simulink model "racing_wheel_lqr_observer"  (R2019b)
settings: Solver=FixedStepAuto  StartTime=0.0  StopTime=inf  FixedStep=0.01  RelTol=1e-3
values from neighbouring files (symbols this model uses):
  Kw = 1/(sys_dis.C*inv(eye(2) - sys_dis.A + sys_dis.B*K)*sys_dis.B)    [controller_LQR_tryout.m]
  P = double([SOL.P1;SOL.P2])    [controller_LQR_tryout.m]
  sys_dis = c2d(sys_con,Ts)    [controller_LQR_tryout.m]
  Ts = 0.02    [controller_LQR_tryout.m]
undefined symbols (not defined in the file or in its folder): K, K_int
libraries: sldrtlib x1
settings Model: EnablePacing=on  Creator=mandl  LastModifiedBy=mandl
settings SolverCC: AlgebraicLoopSolver=LineSearch

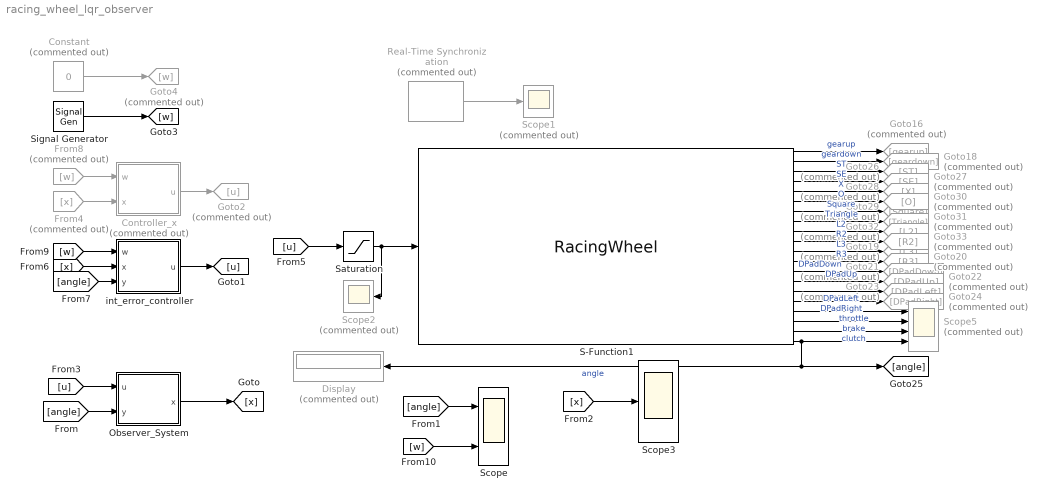
== system racing_wheel_lqr_observer ==
  Constant : Constant  Commented=on  Value=0
  Controller_x : Subsystem  Commented=on
  Display : Display  Commented=on
  From4 : From  Commented=on  GotoTag=x
  From8 : From  Commented=on  GotoTag=w
  Goto16 : Goto  Commented=on  GotoTag=gearup
  Goto18 : Goto  Commented=on  GotoTag=geardown
  Goto19 : Goto  Commented=on  GotoTag=L3
  Goto2 : Goto  Commented=on  GotoTag=u
  Goto20 : Goto  Commented=on  GotoTag=R3
  Goto21 : Goto  Commented=on  GotoTag=DPadDown
  Goto22 : Goto  Commented=on  GotoTag=DPadUp
  Goto23 : Goto  Commented=on  GotoTag=DPadLeft
  Goto24 : Goto  Commented=on  GotoTag=DPadRight
  Goto26 : Goto  Commented=on  GotoTag=ST
  Goto27 : Goto  Commented=on  GotoTag=SE
  Goto28 : Goto  Commented=on  GotoTag=X
  Goto29 : Goto  Commented=on  GotoTag=Square
  Goto30 : Goto  Commented=on  GotoTag=O
  Goto31 : Goto  Commented=on  GotoTag=Triangle
  Goto32 : Goto  Commented=on  GotoTag=L2
  Goto33 : Goto  Commented=on  GotoTag=R2
  Goto4 : Goto  Commented=on  GotoTag=w
  Observer_System : Subsystem
  Real-Time Synchronization : sldrtlib/Real-Time Synchronization  Commented=on  SampleTime=Ts  MaxMissedTicks=inf  ShowMissedTicks=on  YieldWhenWaiting=off
  S-Function1 : S-Function  FunctionName=RacingWheel  Parameters=Ts_FF  SFunctionModules=RacingWheel_wrapper  SFunctionDeploymentMode=off  EnableBusSupport=off  mask(Racing Wheel with Force Feedback){Ts_FF=Ts}
      mask prompts: Ts_FF "Constant Force-Feedback Sample Time"
      mask help: Interacts with the windows gaming API from UWP. The force feedback effect is constant over the user defined sampling time below.
      mask init:
      | val = [[.9  0.75 0.75 1 1 .9 .9 1]',[1 1 0.75 0.75 .9 .9 1 .9]'];try , sys = get_param(gcb,'SfunBuilderFcnName');if isempty(sys), sys = get_param(gcb,'FunctionName'); end,catch, sys = get_param(gcb,'FunctionName'); end
      mask Display:
      | plot(val(:,1),val(:,2)),disp(sys),
      | image('icon.png'),
      | port_label('input',1,'FF'),
      | port_label('output',1,'gearup'),
      | port_label('output',2,'geardown'),
      | port_label('output',3,'ST'),
      | port_label('output',4,'SE'),
      | port_label('output',5,'X'),
      | port_label('output',6,'O'),
      | port_label('output',7,'Square'),
      | port_label('output',8,'Triangle'),
      | port_label('output',9,'L2'),
      | port_label('output',10,'R2'),
      | port_label('output',11,'L3'),
      | port_label('output',12,'R3'),
      | port_label('output',13,'DPadDown'),
      | port_label('output',14,'DPadUp'),
      | port_label('output',15,'DPadLeft'),
      | port_label('output',16,'DPadRight'),
      | port_label('output',17,'throttle'),
      | port_label('output',18,'brake'),
      | port_label('output',19,'clutch'),
      | port_label('output',20,'angle')
  Saturation : Saturate  UpperLimit=1  LowerLimit=-1
  Scope : Scope  NumInputPorts=2
  Scope1 : Scope  Commented=on
  Scope2 : Scope  Commented=on
  Scope3 : Scope
  Scope5 : Scope  Commented=on  NumInputPorts=4
  Signal Generator : SignalGenerator  Amplitude=0.9  Frequency=0.1
  int_error_controller : Subsystem
  wires:
  Real-Time Synchronization/1 -> Scope1/1
  S-Function1/4 -> Goto27/1  "SE"
  S-Function1/17 -> Scope5/1  "throttle"
  S-Function1/5 -> Goto28/1  "X"
  S-Function1/13 -> Goto21/1  "DPadDown"
  S-Function1/8 -> Goto31/1  "Triangle"
  S-Function1/11 -> Goto19/1  "L3"
  S-Function1/10 -> Goto33/1  "R2"
  S-Function1/1 -> Goto16/1  "gearup"
  S-Function1/18 -> Scope5/2  "brake"
  S-Function1/14 -> Goto22/1  "DPadUp"
  S-Function1/3 -> Goto26/1  "ST"
  S-Function1/6 -> Goto30/1  "O"
  S-Function1/7 -> Goto29/1  "Square"
  S-Function1/15 -> Goto23/1  "DPadLeft"
  S-Function1/9 -> Goto32/1  "L2"
  S-Function1/12 -> Goto20/1  "R3"
  S-Function1/2 -> Goto18/1  "geardown"
  S-Function1/19 -> Scope5/3  "clutch"
  S-Function1/16 -> Goto24/1  "DPadRight"
  S-Function1/20 -> Scope5/4, [angle], Display/1  "angle"
  [angle] -> Observer_System/2(y)
  [u] -> Observer_System/1(u)
  From8/1 -> Controller_x/1(w)
  From4/1 -> Controller_x/2(x)
  Controller_x/1(u) -> Goto2/1
  [u] -> Saturation/1
  [angle] -> Scope/1
  Saturation/1 -> Scope2/1, S-Function1/1
  [x] -> Scope3/1
  [x] -> int_error_controller/2(x)
  [w] -> int_error_controller/1(w)
  int_error_controller/1(u) -> [u]
  [angle] -> int_error_controller/3(y)
  Signal Generator/1 -> [w]
  Constant/1 -> Goto4/1
  [w] -> Scope/2
  Observer_System/1(x) -> [x]

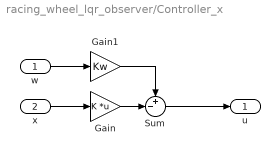
== system racing_wheel_lqr_observer/Controller_x ==
  w : Inport
  x : Inport  Port=2
  Gain : Gain  Gain=K  Multiplication=Matrix(K*u)
  Gain1 : Gain  Gain=Kw
  Sum : Sum  Inputs=+-|
  u : Outport
  wires:
  Gain1/1 -> Sum/1
  Gain/1 -> Sum/2
  x/1 -> Gain/1
  Sum/1 -> u/1
  w/1 -> Gain1/1

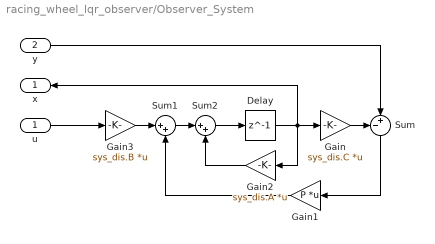
== system racing_wheel_lqr_observer/Observer_System ==
  u : Inport
  y : Inport  Port=2
  Delay : Delay  DelayLength=1  InitialCondition=[0,0]  SampleTime=Ts
  Gain : Gain  Gain=sys_dis.C  Multiplication=Matrix(K*u)
  Gain1 : Gain  Gain=P  Multiplication=Matrix(K*u)
  Gain2 : Gain  Gain=sys_dis.A  Multiplication=Matrix(K*u)
  Gain3 : Gain  Gain=sys_dis.B  Multiplication=Matrix(K*u)
  Sum : Sum  Inputs=-+|
  Sum1 : Sum  Inputs=|++
  Sum2 : Sum  Inputs=|++
  x : Outport
  wires:
  Sum/1 -> Gain1/1
  u/1 -> Gain3/1
  Gain/1 -> Sum/1
  Gain1/1 -> Sum1/2
  Sum1/1 -> Sum2/1
  Delay/1 -> x/1, Gain2/1, Gain/1
  Sum2/1 -> Delay/1
  Gain2/1 -> Sum2/2
  Gain3/1 -> Sum1/1
  y/1 -> Sum/2

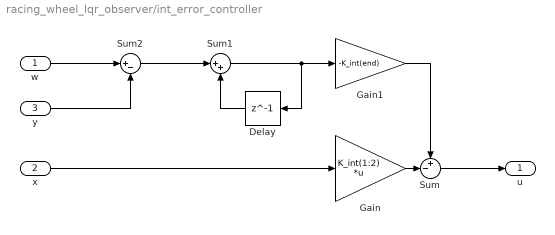
== system racing_wheel_lqr_observer/int_error_controller ==
  w : Inport
  x : Inport  Port=2
  y : Inport  Port=3
  Delay : Delay  DelayLength=1  SampleTime=Ts
  Gain : Gain  Gain=K_int(1:2)  Multiplication=Matrix(K*u)
  Gain1 : Gain  Gain=-K_int(end)
  Sum : Sum  Inputs=+-|
  Sum1 : Sum  Inputs=|++
  Sum2 : Sum  Inputs=|+-
  u : Outport
  wires:
  Gain1/1 -> Sum/1
  Gain/1 -> Sum/2
  x/1 -> Gain/1
  Sum/1 -> u/1
  Sum1/1 -> Delay/1, Gain1/1
  Delay/1 -> Sum1/2
  Sum2/1 -> Sum1/1
  w/1 -> Sum2/1
  y/1 -> Sum2/2
